simulink library "ReceiveFromInputDevice"  (R2016b)
settings: Solver=VariableStepAuto  StartTime=0.0  StopTime=10.0  RelTol=1e-3
settings Model: Creator=Nathan  LastModifiedBy=march

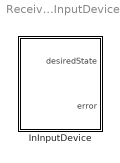
== system ReceiveFromInputDevice ==
  InInputDevice : Subsystem

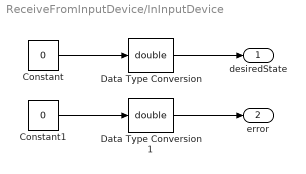
== system ReceiveFromInputDevice/InInputDevice ==
  Constant : Constant  Value=0
  Constant1 : Constant  Value=0
  Data Type Conversion : DataTypeConversion  OutDataTypeStr=double
  Data Type Conversion1 : DataTypeConversion  OutDataTypeStr=double
  desiredState : Outport
  error : Outport  Port=2
  wires:
  Constant1/1 -> Data Type Conversion1/1
  Constant/1 -> Data Type Conversion/1
  Data Type Conversion/1 -> desiredState/1
  Data Type Conversion1/1 -> error/1
